simulink model "untitled3"  (R2019a)
settings: Solver=VariableStepAuto  StartTime=0.0  StopTime=10.0  RelTol=1e-3
libraries: powerlib x7, simulink x1
settings Model: Creator=tiany  LastModifiedBy=tiany

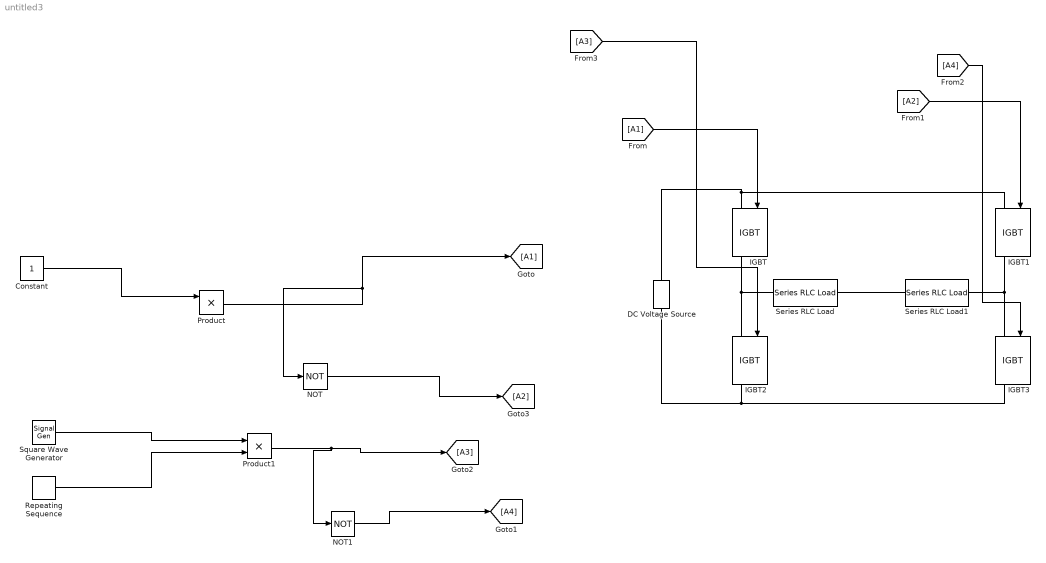
== system untitled3 ==
  Constant : Constant
  DC Voltage Source : powerlib/Electrical Sources/DC Voltage Source  Amplitude=100  Measurements=None
      settings: SourceProductName=Simscape Electrical
  IGBT{,1..3} (4 alike) : powerlib/Power Electronics/IGBT  Ron=0.001  Lon=0  Vf=1  Tf=1e-6  Tt=2e-6  IC=0  Rs=1e5  Cs=inf  Measurements=on
      settings: SourceProductName=Simscape Electrical
  NOT : Logic  Operator=NOT  IconShape=distinctive  AllPortsSameDT=off  OutDataTypeStr=boolean
  NOT1 : Logic  Operator=NOT  IconShape=distinctive  AllPortsSameDT=off  OutDataTypeStr=boolean
  Product : Product
  Product1 : Product
  Repeating Sequence : simulink/Sources/Repeating Sequence  rep_seq_t=[0 2]  rep_seq_y=[0 2]
  Series RLC Load : powerlib/Elements/Series RLC Load  LConnTagsString=a  RConnTagsString=__new0  NominalVoltage=1000  NominalFrequency=60  ActivePower=10e3  InductivePower=100  CapacitivePower=100  Setx0=off  InitialVoltage=0  SetiL0=off  InitialCurrent=0  Measurements=None  LoadType=constant Z
      settings: SourceProductName=Simscape Electrical
  Series RLC Load1 : powerlib/Elements/Series RLC Load  LConnTagsString=a  RConnTagsString=__new0  NominalVoltage=1000  NominalFrequency=60  ActivePower=10e3  InductivePower=100  CapacitivePower=100  Setx0=off  InitialVoltage=0  SetiL0=off  InitialCurrent=0  Measurements=None  LoadType=constant Z
      settings: SourceProductName=Simscape Electrical
  Square Wave Generator : SignalGenerator  WaveForm=square  Units=rad/sec
  wires:
  [A1] -> IGBT/1
  [A3] -> IGBT2/1
  [A2] -> IGBT1/1
  [A4] -> IGBT3/1
  NOT/1 -> [A2]
  NOT1/1 -> [A4]
  Constant/1 -> Product/1
  Product/1 -> NOT/1, [A1]
  Repeating Sequence/1 -> Product1/2
  Square Wave Generator/1 -> Product1/1
  Product1/1 -> NOT1/1, [A3]
  connections:
  DC Voltage Source/RConn1 -- IGBT1/LConn1 -- IGBT/LConn1
  DC Voltage Source/LConn1 -- IGBT3/RConn1 -- IGBT2/RConn1
  IGBT1/RConn1 -- Series RLC Load1/RConn1 -- IGBT3/LConn1
  IGBT/RConn1 -- Series RLC Load/LConn1 -- IGBT2/LConn1
  Series RLC Load/RConn1 -- Series RLC Load1/LConn1
